simulink model "Task2_2_Robust_CBF"  (R2024b)
settings: Solver=ode45  StartTime=0.0  StopTime=30  MaxStep=0.01  RelTol=1e-3
InitFcn:
  | if ~exist('params','var'), params=System_Parameters(); end; if ~exist('simcfg','var'), simcfg=Simulink_Config(params); end;
undefined symbols (not defined in the file): params, simcfg
libraries: simulink_extras x1
settings Model: Creator=LAPTOPASADI  LastModifiedBy=LAPTOPASADI

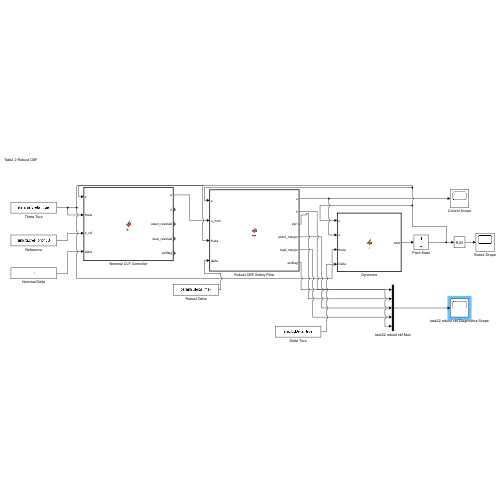
[thumbnail: Simulink's stored preview of the top-level diagram]
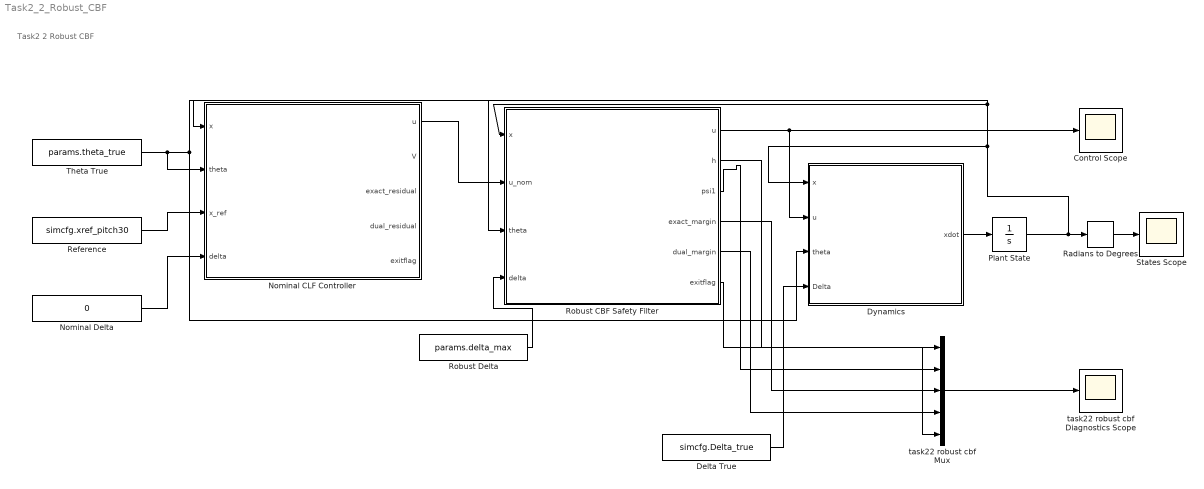
== system Task2_2_Robust_CBF ==
  note: Task2 2 Robust CBF
  Control Scope : Scope
  Delta True : Constant  Value=simcfg.Delta_true
  Dynamics : MATLAB Function  TreatAsAtomicUnit=on
  Nominal CLF Controller : MATLAB Function  TreatAsAtomicUnit=on
  Nominal Delta : Constant  Value=0
  Plant State : Integrator  InitialCondition=simcfg.x0_safe
  Radians to Degrees : simulink_extras/Transformations/Radians to Degrees
  Reference : Constant  Value=simcfg.xref_pitch30
  Robust CBF Safety Filter : MATLAB Function  TreatAsAtomicUnit=on
  Robust Delta : Constant  Value=params.delta_max
  States Scope : Scope
  Theta True : Constant  Value=params.theta_true
  task22 robust cbf Diagnostics Scope : Scope
  task22 robust cbf Mux : Mux  Inputs=5
  wires:
  Plant State/1 -> Radians to Degrees/1, Nominal CLF Controller/1(x), Robust CBF Safety Filter/1(x), Dynamics/1(x)
  Theta True/1 -> Robust CBF Safety Filter/3(theta), Dynamics/3(theta), Nominal CLF Controller/2(theta)
  Reference/1 -> Nominal CLF Controller/3(x_ref)
  Nominal Delta/1 -> Nominal CLF Controller/4(delta)
  Nominal CLF Controller/1(u) -> Robust CBF Safety Filter/2(u_nom)
  Robust Delta/1 -> Robust CBF Safety Filter/4(delta)
  Robust CBF Safety Filter/1(u) -> Control Scope/1, Dynamics/2(u)
  Delta True/1 -> Dynamics/4(Delta)
  Dynamics/1(xdot) -> Plant State/1
  Robust CBF Safety Filter/2(h) -> task22 robust cbf Mux/1
  Robust CBF Safety Filter/3(psi1) -> task22 robust cbf Mux/2
  Robust CBF Safety Filter/4(exact_margin) -> task22 robust cbf Mux/3
  Robust CBF Safety Filter/5(dual_margin) -> task22 robust cbf Mux/4
  Robust CBF Safety Filter/6(exitflag) -> task22 robust cbf Mux/5
  task22 robust cbf Mux/1 -> task22 robust cbf Diagnostics Scope/1
  Radians to Degrees/1 -> States Scope/1

== matlab function Task2_2_Robust_CBF/Robust CBF Safety Filter ==
  data: x input; u output; u_nom input; theta input; delta input; h output; psi1 output; exact_margin output; dual_margin output; exitflag output
function [u,h,psi1,exact_margin,dual_margin,exitflag] = fcn(x,u_nom,theta,delta)
G=[0 0 40.75371832714017 8.6858779355964231;0 5.9859154929577469 0 0;0 0 2.4098880670272087 -9.893830239002293]; theta_max=0.3490658503988659; alpha1=5; alpha2=5;
x=reshape(x,6,1);u_nom=reshape(u_nom,4,1);theta=reshape(theta,6,1);
lower=[-inf;-inf;-inf;-inf];upper=[inf;inf;inf;inf];
[h,psi1,Lf,phi_h,a]=hocbf_terms(x,G,theta_max,alpha1);
drift=Lf+phi_h'*theta; b=drift+alpha2*psi1; beta=delta*norm(a,2);
[u,exitflag]=solve_l1_cbf(u_nom,a,b,beta,lower,upper);
if exitflag<=0
    u=best_effort(u_nom,a,beta,lower,upper);
end
nominal=drift+a*u+alpha2*psi1;
exact_margin=nominal-beta*norm(u,2);
dual_margin=nominal-beta*sum(abs(u));
end

function [h,psi1,Lf,phi_h,Lg]=hocbf_terms(x,G,theta_max,alpha1)
phi=x(1);pitch=x(2);w=x(4:6);
[J,Jphi,Jpitch]=kinematics(phi,pitch);
rates=J*w;Jdot=Jphi*rates(1)+Jpitch*rates(2);
p=x(4);q=x(5);r=x(6);
Fw=[p*q,-q*r,0,0,0,-p;0,0,p*r,-(p^2-r^2),0,-q;-q*r,0,0,0,p*q,-r];
J2=J(2,:);h=theta_max-pitch;psi1=-rates(2)+alpha1*h;
Lf=-Jdot(2,:)*w-alpha1*rates(2);phi_h=(-J2*Fw)';Lg=-J2*G;
end

function [J,Jphi,Jpitch]=kinematics(phi,pitch)
c=cos(phi);s=sin(phi);cp=cos(pitch);
if abs(cp)<1e-6,cp=sign(cp+eps)*1e-6;end
t=sin(pitch)/cp;sec=1/cp;
J=[1,s*t,c*t;0,c,-s;0,s*sec,c*sec];
Jphi=[0,c*t,-s*t;0,-s,-c;0,c*sec,-s*sec];
Jpitch=[0,s*sec^2,c*sec^2;0,0,0;0,s*sec*t,c*sec*t];
end

function [best,flag]=solve_l1_cbf(v,a,b,beta,lower,upper)
tol=1e-10;best=min(max(v,lower),upper);best_cost=inf;flag=-2;
for mask=0:15
    signs=zeros(4,1);
    for j=1:4
        if bitget(mask,j),signs(j)=1;else,signs(j)=-1;end
    end
    lo=lower;hi=upper;positive=signs>0;
    lo(positive)=max(lo(positive),0);hi(~positive)=min(hi(~positive),0);
    if any(lo>hi),continue;end
    row=-a+beta*signs';
    [candidate,ok]=project_point(v,row,b,lo,hi,tol);
    if ok>0 && -a*candidate+beta*sum(abs(candidate))<=b+tol
        cost=sum((candidate-v).^2);
        if cost<best_cost,best=candidate;best_cost=cost;flag=1;end
    end
end
end

function [u,flag]=project_point(v,a,b,lower,upper,tol)
u=min(max(v,lower),upper);
if a*u<=b+tol,flag=1;return;end
umin=u;umin(a>0)=lower(a>0);umin(a<0)=upper(a<0);
if a*umin>b+tol,u=umin;flag=-2;return;end
lo=0;hi=1;
while a*min(max(v-hi*a',lower),upper)>b
    hi=2*hi;if hi>1e12,u=umin;flag=-2;return;end
end
for k=1:70
    mid=0.5*(lo+hi);candidate=min(max(v-mid*a',lower),upper);
    if a*candidate>b,lo=mid;else,hi=mid;end
end
u=min(max(v-hi*a',lower),upper);flag=1;
end

function u=best_effort(v,a,beta,lower,upper)
if any(~isfinite([lower;upper])),u=min(max(v,lower),upper);return;end
u=zeros(4,1);
for j=1:4
    z=min(max(0,lower(j)),upper(j));c=[lower(j);z;upper(j)];
    score=a(j)*c-beta*abs(c);best_score=max(score);
    chosen=c(1);best_distance=inf;
    for k=1:3
        if abs(score(k)-best_score)<=1e-14
            distance=abs(c(k)-v(j));
            if distance<best_distance,chosen=c(k);best_distance=distance;end
        end
    end
    u(j)=chosen;
end
end

== matlab function Task2_2_Robust_CBF/Nominal CLF Controller ==
  data: x input; u output; theta input; x_ref input; delta input; V output; exact_residual output; dual_residual output; exitflag output
function [u,V,exact_residual,dual_residual,exitflag] = fcn(x,theta,x_ref,delta)
P=[0.11250000000000002 0 0 0.012500000000000001 0 0;0 0.11250000000000002 0 0 0.012500000000000001 0;0 0 0.11250000000000002 0 0 0.012500000000000001;0.012500000000000001 0 0 0.015625 0 0;0 0.012500000000000001 0 0 0.015625 0;0 0 0.012500000000000001 0 0 0.015625]; G=[0 0 40.75371832714017 8.6858779355964231;0 5.9859154929577469 0 0;0 0 2.4098880670272087 -9.893830239002293]; gamma=0.5;
x=reshape(x,6,1);theta=reshape(theta,6,1);x_ref=reshape(x_ref,6,1);
lower=[-inf;-inf;-inf;-inf]; upper=[inf;inf;inf;inf];
[V,omega,phiV,a]=clf_terms(x,x_ref,P,G);
drift=omega+phiV'*theta;
b=-gamma*V-drift;
beta=delta*norm(a,2);
[u,exitflag]=solve_l1(a,b,beta,lower,upper);
if exitflag<=0
    [u,exitflag]=solve_spectral(a,b,beta,lower,upper);
end
dual_residual=drift+a*u+beta*sum(abs(u))+gamma*V;
exact_residual=drift+a*u+beta*norm(u,2)+gamma*V;
end

function [V,omega,phiV,LgV]=clf_terms(x,x_ref,P,G)
phi=x(1); pitch=x(2); w=x(4:6);
[J,Jphi,Jpitch]=kinematics(phi,pitch);
rates=J*w; Jdot=Jphi*rates(1)+Jpitch*rates(2);
eta=[x(1:3)-x_ref(1:3);rates];
p=x(4);q=x(5);r=x(6);
Fw=[p*q,-q*r,0,0,0,-p;0,0,p*r,-(p^2-r^2),0,-q;-q*r,0,0,0,p*q,-r];
grad=2*P*eta; V=eta'*P*eta;
omega=grad(1:3)'*rates+grad(4:6)'*(Jdot*w);
phiV=(J*Fw)'*grad(4:6); LgV=grad(4:6)'*(J*G);
end

function [J,Jphi,Jpitch]=kinematics(phi,pitch)
c=cos(phi);s=sin(phi);cp=cos(pitch);
if abs(cp)<1e-6,cp=sign(cp+eps)*1e-6;end
t=sin(pitch)/cp;sec=1/cp;
J=[1,s*t,c*t;0,c,-s;0,s*sec,c*sec];
Jphi=[0,c*t,-s*t;0,-s,-c;0,c*sec,-s*sec];
Jpitch=[0,s*sec^2,c*sec^2;0,0,0;0,s*sec*t,c*sec*t];
end

function [best,flag]=solve_l1(a,b,beta,lower,upper)
tol=1e-10; best=zeros(4,1); best_cost=inf; flag=-2;
unbounded=all(isinf(lower)&lower<0)&&all(isinf(upper)&upper>0);
for mask=0:15
    signs=zeros(4,1);
    for j=1:4
        if bitget(mask,j),signs(j)=1;else,signs(j)=-1;end
    end
    lo=lower;hi=upper;positive=signs>0;
    lo(positive)=max(lo(positive),0);hi(~positive)=min(hi(~positive),0);
    if any(lo>hi),continue;end
    row=a+beta*signs';
    if unbounded
        if b>=-tol
            candidate=zeros(4,1);ok=1;
        else
            direction=-row';direction(signs.*direction<0)=0;
            denominator=row*direction;
            if denominator<-eps,candidate=(b/denominator)*direction;ok=1;
            else,candidate=zeros(4,1);ok=-2;end
        end
    else
        [candidate,ok]=project_origin(row,b,lo,hi,tol);
    end
    if ok>0 && a*candidate+beta*sum(abs(candidate))<=b+tol
        cost=candidate'*candidate;
        if cost<best_cost,best=candidate;best_cost=cost;flag=1;end
    end
end
end

function [u,flag]=project_origin(a,b,lower,upper,tol)
u=min(max(zeros(4,1),lower),upper);
if a*u<=b+tol,flag=1;return;end
umin=u;umin(a>0)=lower(a>0);umin(a<0)=upper(a<0);
if a*umin>b+tol,u=umin;flag=-2;return;end
lo=0;hi=1;
while a*min(max(-hi*a',lower),upper)>b
    hi=2*hi;if hi>1e12,u=umin;flag=-2;return;end
end
for k=1:80
    mid=0.5*(lo+hi);candidate=min(max(-mid*a',lower),upper);
    if a*candidate>b,lo=mid;else,hi=mid;end
end
u=min(max(-hi*a',lower),upper);flag=1;
end

function [u,flag]=solve_spectral(a,b,beta,lower,upper)
tol=1e-10;u=min(max(zeros(4,1),lower),upper);
if a*u+beta*norm(u)<=b+tol,flag=1;return;end
lo=0;hi=1;previous=nan(4,1);
while true
    candidate=min(max(-hi*a',lower),upper);
    if a*candidate+beta*norm(candidate)<=b+tol,break;end
    if all(isfinite(previous))&&norm(candidate-previous,inf)<=eps,u=candidate;flag=-2;return;end
    previous=candidate;hi=2*hi;
    if hi>1e12,u=candidate;flag=-2;return;end
end
for k=1:80
    mid=0.5*(lo+hi);candidate=min(max(-mid*a',lower),upper);
    if a*candidate+beta*norm(candidate)>b,lo=mid;else,hi=mid;end
end
u=min(max(-hi*a',lower),upper);flag=1;
end

== matlab function Task2_2_Robust_CBF/Dynamics ==
  data: x input; u input; xdot output; theta input; Delta input
function xdot = fcn(x,u,theta,Delta)
G = [0 0 40.75371832714017 8.6858779355964231;0 5.9859154929577469 0 0;0 0 2.4098880670272087 -9.893830239002293];
x=reshape(x,6,1);
u=reshape(u,4,1);
theta=reshape(theta,6,1);
Delta=reshape(Delta,4,4);

phi = x(1);
pitch = x(2);
p = x(4);
q = x(5);
r = x(6);

cphi = cos(phi);
sphi = sin(phi);
cpitch = cos(pitch);
if abs(cpitch) < 1e-6
    cpitch = sign(cpitch+eps)*1e-6;
end
tpitch = sin(pitch)/cpitch;

J = [1, sphi*tpitch, cphi*tpitch;
     0, cphi,         -sphi;
     0, sphi/cpitch,  cphi/cpitch];
f0 = [J*[p;q;r]; zeros(3,1)];
Fomega = [p*q, -q*r, 0, 0, 0, -p;
          0, 0, p*r, -(p^2-r^2), 0, -q;
          -q*r, 0, 0, 0, p*q, -r];
F = [zeros(3,6); Fomega];
g = [zeros(3,4); G];
xdot = f0+F*theta+g*(eye(4)+Delta)*u;
end
